simulink model "projeto_garra_3"  (R2024b)
settings: Solver=FixedStepAuto  StartTime=0.0  StopTime=10.0  RelTol=1e-3
model workspace (MAT data in the model file):
  SL_ROS_VariableLengthArrays_MaxSizes.CommonInfo.ArrayTruncateAction = 'EmitWarning'
  SL_ROS_VariableLengthArrays_MaxSizes.MsgTypeMap = containers.Map
  SL_ROS_VariableLengthArrays_MaxSizes.MsgTypeMap.serialization.keys = {'sensor_msgs/Image', 'trajectory_msgs/JointTrajectory'}
  SL_ROS_VariableLengthArrays_MaxSizes.MsgTypeMap.serialization.values{1}(1).PropertyName = 'Data'
  SL_ROS_VariableLengthArrays_MaxSizes.MsgTypeMap.serialization.values{1}(1).DataType = 'uint8'
  SL_ROS_VariableLengthArrays_MaxSizes.MsgTypeMap.serialization.values{1}(1).MaxLength = 1228800
  SL_ROS_VariableLengthArrays_MaxSizes.MsgTypeMap.serialization.values{1}(2).PropertyName = 'Encoding'
  SL_ROS_VariableLengthArrays_MaxSizes.MsgTypeMap.serialization.values{1}(2).DataType = 'uint8'
  SL_ROS_VariableLengthArrays_MaxSizes.MsgTypeMap.serialization.values{1}(2).MaxLength = 128
  SL_ROS_VariableLengthArrays_MaxSizes.MsgTypeMap.serialization.values{2}(1).PropertyName = 'JointNames'
  SL_ROS_VariableLengthArrays_MaxSizes.MsgTypeMap.serialization.values{2}(1).DataType = 'std_msgs/String'
  SL_ROS_VariableLengthArrays_MaxSizes.MsgTypeMap.serialization.values{2}(1).MaxLength = 16
  SL_ROS_VariableLengthArrays_MaxSizes.MsgTypeMap.serialization.values{2}(2).PropertyName = 'Points'
  SL_ROS_VariableLengthArrays_MaxSizes.MsgTypeMap.serialization.values{2}(2).DataType = 'trajectory_msgs/JointTrajectoryPoint'
  SL_ROS_VariableLengthArrays_MaxSizes.MsgTypeMap.serialization.values{2}(2).MaxLength = 7
  SL_ROS_VariableLengthArrays_MaxSizes.MsgTypeMap.serialization.uniformity = 0
  SL_ROS_VariableLengthArrays_MaxSizes.MsgTypeMap.serialization.keyType = 'char'
  SL_ROS_VariableLengthArrays_MaxSizes.MsgTypeMap.serialization.valueType = 'any'
libraries: robotlib x8
settings Model: ExtModeBatchMode=on  Creator=pecci  LastModifiedBy=roboime
settings OptimizationCC: DefaultParameterBehavior=Inlined  EnhancedBackFolding=on  PassReuseOutputArgsAs=Individual arguments  ZeroExternalMemoryAtStartup=off  ZeroInternalMemoryAtStartup=off  MaxStackSize=64  OptimizeBlockOrder=speed  DifferentSizesBufferReuse=on  OptimizationCustomize=off  EfficientTunableParamExpr=on
settings DebuggingCC: ParameterTunabilityLossMsg=error
settings HardwareCC: ProdBitPerPointer=32  ProdBitPerSizeT=32  ProdBitPerPtrDiffT=32  ProdLargestAtomicFloat=None  ProdIntDivRoundTo=Undefined  ProdEndianess=Unspecified  ProdWordSize=32  ProdHWDeviceType=Generic->Unspecified (assume 32-bit Generic)
settings SFSimCC: MATLABDynamicMemAlloc=off
settings RTWCC: Description=Embedded Coder  SystemTargetFile=ert.tlc  HardwareBoard=Robot Operating System (ROS)  TLCOptions="-aInlineSetEventsForThisBaseRateFcn=TLC_FALSE -aSuppressMultiTaskScheduler=TLC_FALSE  -aRateBasedStepFcn=0"  TemplateMakefile=ert_default_tmf  Toolchain=Catkin  TargetLang=C++
settings CodeAppCC: ForceParamTrailComments=on  IgnoreCustomStorageClasses=off  OperatorAnnotations=on  SimulinkDataObjDesc=on  SFDataObjDesc=on  InsertBlockDesc=on

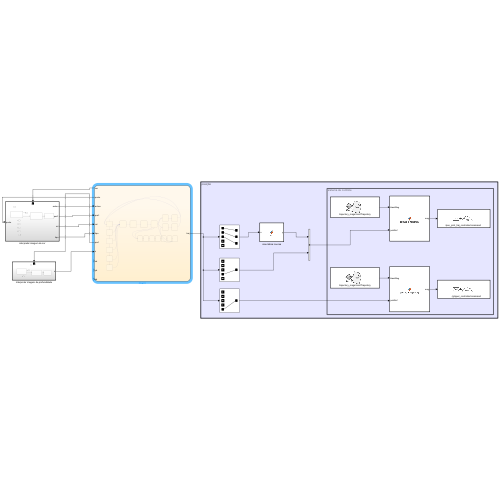
[thumbnail: Simulink's stored preview of the top-level diagram]
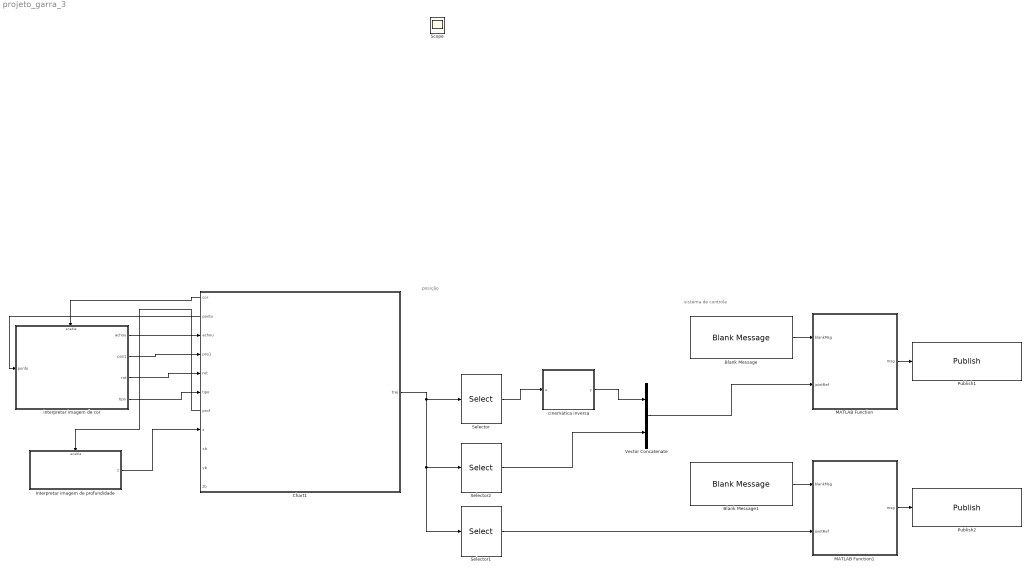
== system projeto_garra_3 ==
  note: posição
  note: sistema de controle
  Blank Message : robotlib/Blank Message  messageClass=Message  entityType=trajectory_msgs/JointTrajectory  messageType=trajectory_msgs/JointTrajectory  SampleTime=inf  legacyBusStruct=off
  Blank Message1 : robotlib/Blank Message  messageClass=Message  entityType=trajectory_msgs/JointTrajectory  messageType=trajectory_msgs/JointTrajectory  SampleTime=inf  legacyBusStruct=off
  Chart1 : Stateflow chart  TreatAsAtomicUnit=on
      settings: PortSchema="{\"entries\":[{\"content\":{\"sides\":[{\"content\":{\"connectorIds\":[\"Out1\",\"Out4\",\"In1\",\"In2\",\"In3\",\"In4\",\"Out2\",\"In5\",\"In6\",\"In7\",\"In8\"]},\"type\":\"ConnectorPlacement.EquallySpacedRectSide\",\"uuid\":\"2ce0c57c-c8af-493e-b7a7-7a5f5fd3398e\"},{\"content\":{\"connectorIds\":[\"Out3\"],\"side\":\"RIGHT\"},\"type\":\"ConnectorPlacement.EquallySpacedRectSide\",\"uuid\":\"3b5d3580-bb24-4e36-a1dd-ff8ebdeb0e78\"},{\"content\":{\"side\":\"TOP\"},\"type\":\"ConnectorPlacement.EquallySpacedRectSide\",\"uuid\":\"3bc7b972-0a1c-463f-be80-f32afe00e7c2\"}]},\"type\":\"ConnectorPlacement.EquallySpacedConnector\",\"uuid\":\"b1a750b7-98c0-4bfd-8e60-8f2b1050b174\"}],\"packageUris\":[\"http://schema.mathworks.com/mf0/Connector/R2020b\"],\"version\":\"1.0\"}"
  Interpretar imagem de profundidade : Subsystem
  MATLAB Function : MATLAB Function  TreatAsAtomicUnit=on
  MATLAB Function1 : MATLAB Function  TreatAsAtomicUnit=on
  Publish1 : robotlib/Publish  topicSource=Select from ROS network  topic=/pos_joint_traj_controller/command  messageType=trajectory_msgs/JointTrajectory  legacyBusStruct=off  messageQueueLength=1
  Publish2 : robotlib/Publish  topicSource=Select from ROS network  topic=/gripper_controller/command  messageType=trajectory_msgs/JointTrajectory  legacyBusStruct=off  messageQueueLength=1
  Selector : Selector  InputPortWidth=5  IndexOptions=Index vector (dialog)  Indices=[1 2 3]  OutputSizes=1
  Selector1 : Selector  InputPortWidth=5  IndexOptions=Index vector (dialog)  Indices=[5]  OutputSizes=1
  Selector2 : Selector  InputPortWidth=5  IndexOptions=Index vector (dialog)  Indices=[4]  OutputSizes=1
  Vector Concatenate : Concatenate
  cinemática inversa : MATLAB Function  TreatAsAtomicUnit=on
  interpretar imagem de cor : Subsystem
  Scope : Scope
  wires:
  Chart1/3(traj) -> Selector1/1, Selector2/1, Selector/1
  Selector1/1 -> MATLAB Function1/2(jointRef)
  Selector2/1 -> Vector Concatenate/2
  Selector/1 -> cinemática inversa/1(u)
  cinemática inversa/1(y) -> Vector Concatenate/1
  Blank Message1/1 -> MATLAB Function1/1(blankMsg)
  Blank Message/1 -> MATLAB Function/1(blankMsg)
  MATLAB Function/1(msg) -> Publish1/1
  Vector Concatenate/1 -> MATLAB Function/2(jointRef)
  MATLAB Function1/1(msg) -> Publish2/1
  Chart1/1(cor) -> interpretar imagem de cor/Enable
  Chart1/2(prof) -> Interpretar imagem de profundidade/Enable
  Interpretar imagem de profundidade/1(z) -> Chart1/5(z)
  interpretar imagem de cor/4(tipo) -> Chart1/4(tipo)
  interpretar imagem de cor/3(rot) -> Chart1/3(rot)
  interpretar imagem de cor/2(pos1) -> Chart1/2(pos1)
  interpretar imagem de cor/1(achou) -> Chart1/1(achou)
  Chart1/4(ponto) -> interpretar imagem de cor/1(ponto)

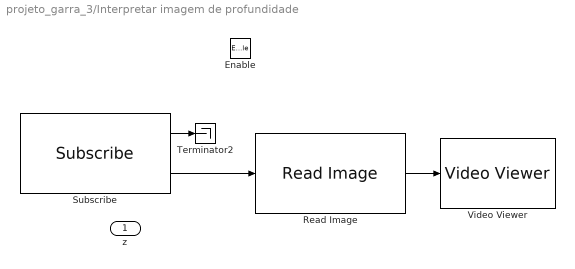
== system projeto_garra_3/Interpretar imagem de profundidade ==
  Enable : EnablePort
  Read Image : robotlib/Read Image  MaximumImageSize=[480, 640]  ImageEncoding=32fc1  ShowAlphaOutput=off  ShowErrorCodeOutput=off  VariableSizeOutputs=off
  Subscribe : robotlib/Subscribe  topicSource=Select from ROS network  topic=/camera/depth/image_raw  messageType=sensor_msgs/Image  SampleTime=1  legacyBusStruct=off  messageQueueLength=1
  Terminator2 : Terminator
  Video Viewer : VideoViewer  FigPos=[795 440 418 304]
  z : Outport
  wires:
  Read Image/1 -> Video Viewer/1
  Subscribe/2 -> Read Image/1
  Subscribe/1 -> Terminator2/1

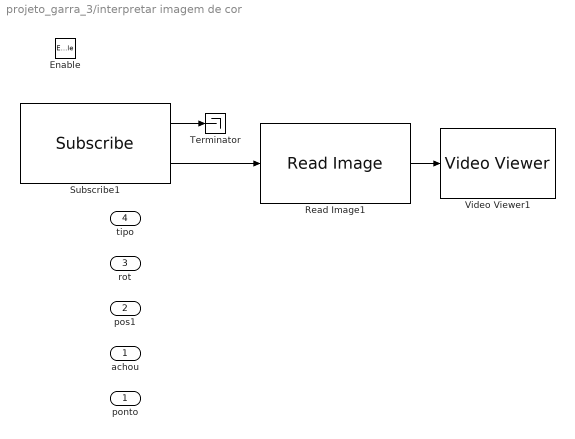
== system projeto_garra_3/interpretar imagem de cor ==
  ponto : Inport
  Enable : EnablePort
  Read Image1 : robotlib/Read Image  MaximumImageSize=[480, 640]  ImageEncoding=bgr8  ShowAlphaOutput=off  ShowErrorCodeOutput=off  VariableSizeOutputs=off
  Subscribe1 : robotlib/Subscribe  topicSource=Select from ROS network  topic=/camera/rgb/image_raw  messageType=sensor_msgs/Image  SampleTime=1  legacyBusStruct=off  messageQueueLength=1
  Terminator : Terminator
  Video Viewer1 : VideoViewer  FigPos=[724 558 418 304]
  achou : Outport
  pos1 : Outport  Port=2
  rot : Outport  Port=3
  tipo : Outport  Port=4
  wires:
  Subscribe1/2 -> Read Image1/1
  Subscribe1/1 -> Terminator/1
  Read Image1/1 -> Video Viewer1/1

== matlab function projeto_garra_3/MATLAB Function1 ==
  data: blankMsg input; msg output Bus: SL_Bus_projeto_garra_2_trajectory_msgs_JointTrajectory; jointRef input
function msg = packageTrajectory(blankMsg, jointRef)

    msg = blankMsg;

    
    numJoints = uint32(1);
    msg.JointNames_SL_Info.CurrentLength = numJoints;

  
    name = 'robotiq_85_left_knuckle_joint';
    msg.JointNames(1).Data(1:length(name)) = uint8(name);
    msg.JointNames(1).Data_SL_Info.CurrentLength = uint32(length(name));

    msg.Points_SL_Info.CurrentLength = uint32(1);

    msg.Points(1).TimeFromStart.Sec = 1;
    msg.Points(1).TimeFromStart.Nsec = 0;

    msg.Points(1).Positions_SL_Info.CurrentLength = numJoints;
    msg.Points(1).Positions(1:numJoints) = jointRef;

    msg.Points(1).Velocities_SL_Info.CurrentLength = numJoints;
    msg.Points(1).Velocities(1:numJoints) = zeros(numJoints,1);

    msg.Points(1).Accelerations_SL_Info.CurrentLength = numJoints;
    msg.Points(1).Accelerations(1:numJoints) = zeros(numJoints,1);

    msg.Points(1).Effort_SL_Info.CurrentLength = numJoints;
    msg.Points(1).Effort(1:numJoints) = zeros(numJoints,1);

    % Header com valores padrão
msg.Header.Stamp.Sec = 0;
msg.Header.Stamp.Nsec = 0;
msg.Header.Seq = uint32(1);
msg.Header.FrameId = uint8(zeros(128,1));  % força 1x128 com transposição
msg.Header.FrameId_SL_Info.CurrentLength = uint32(0);


end

== matlab function projeto_garra_3/MATLAB Function ==
  data: blankMsg input; msg output Bus: SL_Bus_projeto_garra_2_trajectory_msgs_JointTrajectory; jointRef input
function msg = packageTrajectory(blankMsg, jointRef)

    msg = blankMsg;

msg.JointNames_SL_Info.CurrentLength = uint32(6);

msg.JointNames(1).Data_SL_Info.CurrentLength = uint32(18);
msg.JointNames(1).Data(1:18) = uint8('shoulder_pan_joint')';
msg.JointNames(2).Data_SL_Info.CurrentLength = uint32(19);
msg.JointNames(2).Data(1:19) = uint8('shoulder_lift_joint')';
msg.JointNames(3).Data_SL_Info.CurrentLength = uint32(11);
msg.JointNames(3).Data(1:11) = uint8('elbow_joint')';
msg.JointNames(4).Data_SL_Info.CurrentLength = uint32(13);
msg.JointNames(4).Data(1:13) = uint8('wrist_1_joint')';
msg.JointNames(5).Data_SL_Info.CurrentLength = uint32(13);
msg.JointNames(5).Data(1:13) = uint8('wrist_2_joint')';
msg.JointNames(6).Data_SL_Info.CurrentLength = uint32(13);
msg.JointNames(6).Data(1:13) = uint8('wrist_3_joint')';

numJoints = uint32(6);

    msg.Points_SL_Info.CurrentLength = uint32(1);

    msg.Points(1).TimeFromStart.Sec = 1;
    msg.Points(1).TimeFromStart.Nsec = 0;

    msg.Points(1).Positions_SL_Info.CurrentLength = numJoints;
    msg.Points(1).Positions(1:numJoints) = jointRef;

    msg.Points(1).Velocities_SL_Info.CurrentLength = numJoints;
    msg.Points(1).Velocities(1:numJoints) = zeros(numJoints,1);

    msg.Points(1).Accelerations_SL_Info.CurrentLength = numJoints;
    msg.Points(1).Accelerations(1:numJoints) = zeros(numJoints,1);

    msg.Points(1).Effort_SL_Info.CurrentLength = numJoints;
    msg.Points(1).Effort(1:numJoints) = zeros(numJoints,1);

    % Header com valores padrão
msg.Header.Stamp.Sec = 0;
msg.Header.Stamp.Nsec = 0;
msg.Header.Seq = uint32(1);
msg.Header.FrameId = uint8(zeros(128,1));  % força 1x128 com transposição
msg.Header.FrameId_SL_Info.CurrentLength = uint32(0);

end

== stateflow chart projeto_garra_3/Chart1 ==
  state lixeira_verde
    traj(1) = xlv;
    traj(2) = ylv;
    traj(3) = zp;
    traj(4) =0;
    traj(5) =1;
    exit:traj;
  state soltar
    traj(1) = xlv;
    traj(2) = ylv;
    traj(3) = zp;
    traj(4) =0;
    traj(5) =0;
    exit:traj;
  state Posicionar
    entry: pos1(1:2);
    entry: rot;
    traj(1:5);
    traj(1) = pos1(1);
    traj(2) = pos1(2);
    traj(3) = zp;
    traj(4) =rot;
    traj(5) =0;
    exit:traj;
  state Profundidade
    exit:prof = 1
    entry:z;
    traj(1) = pos1(1);
    traj(2) = pos1(2);
    traj(3) = z;
    traj(4) =rot;
    traj(5) =0;
    exit:traj;
  state Pegar
    exit:prof = 1
    entry:z;
    traj(1) = pos1(1);
    traj(2) = pos1(2);
    traj(3) = z;
    traj(4) =rot;
    traj(5) =1;
    exit:traj;
  state Posicionar1
    traj(1) = pos1(1);
    traj(2) = pos1(2);
    traj(3) = zp;
    traj(4) =rot;
    traj(5) =1;
    exit:traj;
    entry:tipo;
  state PP1
    exit:cor = 1;
    exit:ponto = [0,0,0];
    exit:traj = ponto
    entry:achou;
  state lixeira_verde1
    traj(1) = xla;
    traj(2) = yla;
    traj(3) = zp;
    traj(4) =0;
    traj(5) =1;
    exit:traj;
  state soltar1
    traj(1) = xla;
    traj(2) = yla;
    traj(3) = zp;
    traj(4) =0;
    traj(5) =0;
    exit:traj;
  state PP2
    exit:cor = 1;
    exit:ponto = [0,0,0];
    exit:traj = ponto
    entry:achou;
  state balanca
    traj(1) = xb;
    traj(2) = yb;
    traj(3) = zp;
    traj(4) =rot;
    traj(5) =1;
    exit:traj;
    entry:tipo;
  state balanca1
    traj(1) = xb;
    traj(2) = yb;
    traj(3) = zb;
    traj(4) =rot;
    traj(5) =1;
    exit:traj;
    entry:tipo;
  state balanca2
    traj(1) = xb;
    traj(2) = yb;
    traj(3) = zb;
    traj(4) =rot;
    traj(5) =0;
    exit:traj;
    entry:tipo;
  state balanca3
    traj(1) = xb;
    traj(2) = yb;
    traj(3) = zp;
    traj(4) =rot;
    traj(5) =0;
    exit:traj;
    entry:tipo;
  state balanca4
    traj(1) = xb;
    traj(2) = yb;
    traj(3) = zb;
    traj(4) =rot;
    traj(5) =0;
    exit:traj;
    entry:tipo;
  state balanca5
    traj(1) = xb;
    traj(2) = yb;
    traj(3) = zb;
    traj(4) =rot;
    traj(5) =1;
    exit:traj;
    entry:tipo;
  state balanca6
    traj(1) = xb;
    traj(2) = yb;
    traj(3) = zp;
    traj(4) =rot;
    traj(5) =1;
    exit:traj;
    entry:tipo;
  state PP3
    exit:cor = 1;
    exit:ponto = [0,0,0];
    exit:traj = ponto
    entry:achou;
  state PP4
    exit:cor = 1;
    exit:ponto = [0,0,0];
    exit:traj = ponto
    entry:achou;
  state PP5
    exit:cor = 1;
    exit:ponto = [0,0,0];
    exit:traj = ponto
    entry:achou;
  state PP6
    exit:cor = 1;
    exit:ponto = [0,0,0];
    exit:traj = ponto
    entry:achou;
  soltar1 -> PP1
  soltar -> PP1
  Posicionar1 -> lixeira_verde [order 1] : [tipo == 1]
  balanca6 -> lixeira_verde [order 1] : [tipo == 3]
  lixeira_verde -> soltar : after(10,sec)
  (default) -> PP1
  PP1 -> Posicionar [order 2] : [achou == 1]
  Posicionar -> Profundidade : after(10,sec)
  Pegar -> Posicionar1 : after(10,sec)
  Posicionar1 -> lixeira_verde1 [order 2] : [tipo == 2]
  Profundidade -> Pegar : after(10,sec)
  PP2 -> Posicionar [order 2] : [achou == 1]
  PP3 -> Posicionar [order 2] : [achou == 1]
  PP4 -> Posicionar [order 2] : [achou == 1]
  PP5 -> Posicionar [order 2] : [achou == 1]
  PP6 -> Posicionar : [achou == 1]
  PP1 -> PP2 [order 1] : [achou == 0]
  balanca6 -> lixeira_verde1 [order 2] : [tipo == 4]
  lixeira_verde1 -> soltar1 : after(10,sec)
  Posicionar1 -> balanca [order 3] : [tipo == 3]
  Posicionar1 -> balanca [order 4] : [tipo == 4]
  PP2 -> PP3 [order 1] : [achou == 0]
  balanca -> balanca1
  balanca1 -> balanca2
  balanca2 -> balanca3
  balanca3 -> balanca4
  balanca4 -> balanca5
  balanca5 -> balanca6
  PP3 -> PP4 [order 1] : [achou == 0]
  PP4 -> PP5 [order 1] : [achou == 0]
  PP5 -> PP6 [order 1] : [achou == 0]
  data: achou input; pos1 input; cor output; prof output; rot input; tipo input; z input; ylv local; yla local; xla local; xlv local; traj output; ponto output; xb input; yb input; zb input; zp local

== matlab function projeto_garra_3/cinemática inversa ==
  data: u input; y output
function y = fcn(u)

y = u;
